simulink model "testemplanner_cs"  (R2020a)
settings: Solver=ode5  StartTime=0.0  StopTime=24  FixedStep=1/1000  RelTol=1e-3
PreLoadFcn:
  | mbxruntime.callbacks.PreLoadFcn(bdroot);
PostLoadFcn:
  | mbxruntime.callbacks.PostLoadFcn(bdroot);
InitFcn:
  | mbxruntime.callbacks.InitFcn(bdroot);
StartFcn:
  | mbxruntime.callbacks.StartFcn(bdroot);
StopFcn:
  | mbxruntime.callbacks.StopFcn(bdroot);
model workspace (MAT data in the model file):
  mbox_table : object (value not decoded)
  model_closed = 0
  sim_status = 0
values from neighbouring files (symbols this model uses):
  c_factor = 43.75    [emplanner_init.m]
  cf = -175016    [emplanner_init.m]
  cr = -130634    [emplanner_init.m]
  global_path_x = [0.057304 1.05668625507 2.05480936558 3.05165624935 4.04722112279 5.04150235808 6.03449985569 7.02621407764 8.01664569183 9.00579544113 9.99366409523 10.9802524329 ... (3001 elements, 3001x1)]    [global_path.mat]
  global_path_y = [8.29 8.29 8.29 8.29 8.29 8.29 8.29 8.29 8.29 8.29 8.29 8.29 ... (3001 elements, 3001x1)]    [global_path.mat]
  KD_PID_distance = 0.0    (= 0)    [emplanner_init.m]
  KD_PID_speed = 0    [emplanner_init.m]
  KI_PID_distance = 0.0    (= 0)    [emplanner_init.m]
  KI_PID_speed = 0    [emplanner_init.m]
  KP_PID_distance = 0.5    [emplanner_init.m]
  KP_PID_speed = 1.8    [emplanner_init.m]
  la = 1.265    [emplanner_init.m]
  lb = 2.947-1.265    (= 1.682)    [emplanner_init.m]
  LQR_K1 = k(:,1)'    [emplanner_init.m]
  LQR_K2 = k(:,2)'    [emplanner_init.m]
  LQR_K3 = k(:,3)'    [emplanner_init.m]
  LQR_K4 = k(:,4)'    [emplanner_init.m]
  m = 2020    [emplanner_init.m]
  rack_displacement = [-39.14 , -37.2 , -35.29 , -33.43 , -31.6 , -29.81 , -28.06 , -26.34 , -24.66 ,      -23.01 , -21.38 , -19.79 , -18.23 , -16.69 , -15.18 , -13.7 , -12.23 , -10.8 , -9.38 , -7.98 ,     -6.61 , -5.25 , -3.91 , -2.59 , -1.29 , 0 , 1.27 , 2.54 , 3.78 , 5.02 , 6.24 , 7.46 , 8.66 ,      9.86 , 11.05 , 12.24 , 13.41 , 14.59 , 15.76 , 16.92 , 18.09 , 19.25 , 20.42 , 21.59 , 22.76 ,      23.93 , 25.11 , 26 ...(+26 chars)    [emplanner_init.m]
  right_wheel_ground = [-70 ,-67.2 , -64.4 , -61.6 , -58.8 , -56 , -53.2 , -50.4 , -47.6 , -44.8 , -42 ,      -39.2 , -36.4 , -33.6 , -30.8 , -28 , -25.2 , -22.4 , -19.6 , -16.8 , -14 , -11.2 , -8.4 , -5.6 ,      -2.8 , 0 , 2.8 , 5.6 , 8.4 , 11.2 , 14 , 16.8 , 19.6 , 22.4 , 25.2 , 28 , 30.8 , 33.6 , 36.4 ,      39.2 , 42 , 44.8 , 47.6 , 50.4 , 53.2 , 56 , 58.8 , 61.6 , 64.4 , 67.2 , 70 ]    [emplanner_init.m]
  vx_break_point = zeros(1,5000)    [emplanner_init.m]
undefined symbols (not defined in the file or in its folder): aubr, DiscIntNeverNeededParam, tablebr, vubr
libraries: PreScanSimulinkLibrary x9, Solver_SF x1, simulink_extras x1
(part 3 of 9)

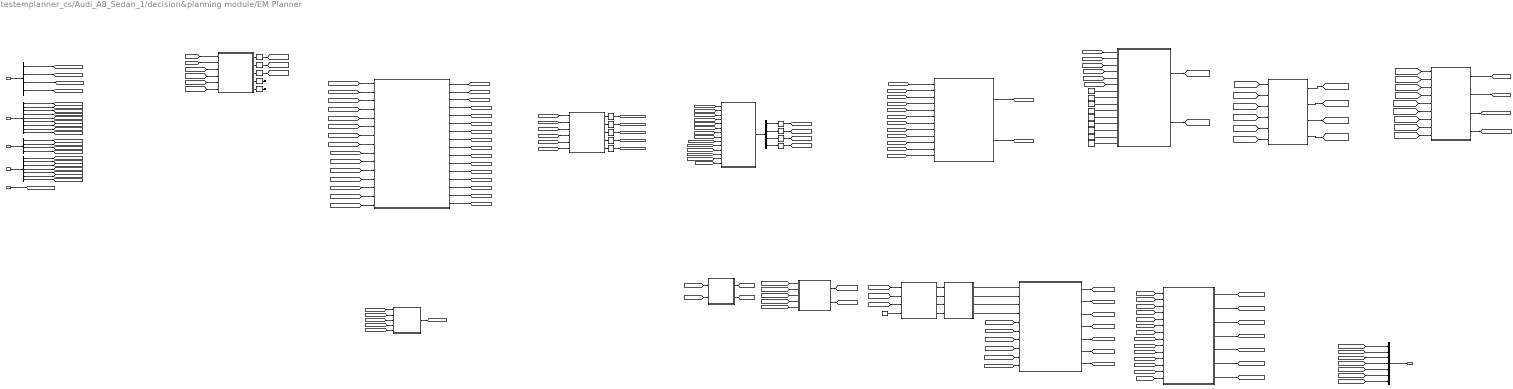
== system testemplanner_cs/Audi_A8_Sedan_1/decision&planning module/EM Planner ==
  note: 计算规划起点的投影点
  note: 模块输入整理，输入包括车辆当前位置、航向、速度、加速度信息。参考线信息，车辆在参考线上的投影点信息，感知获取的障碍物信息，当前的时间戳以及上一周期规划出的路径相关信息
  note: 找到规划路径起点，并通过拼接的方式进行平滑
  note: 计算index对应的s，并形成数组，方便进行查阅
  note: 进行动态规划所求路径的加密，以适应控制的需要
  note: 坐标变换，从Frenet坐标转换为直角坐标，进行控制
  note: 动态规划主函数
  note: 对障碍物进行筛选和投影
  note: 笛卡尔坐标转Frenet坐标
  note: 轨迹生成模块
  referenceline info : Inport
  location info : Inport  Port=2
  perception info : Inport  Port=3
  pre_planning info : Inport  Port=4
  current time : Inport  Port=5
  Bus Creator : BusCreator  Inputs=7
  Bus Selector : BusSelector  OutputSignals=referenceline_x,referenceline_y,path_heading,path_kappa
  Bus Selector1 : BusSelector  OutputSignals=host_x,host_y,host_heading_xy,host_vx,host_vy,host_yawrate,host_speed,host_ax,host_ay
  Bus Selector2 : BusSelector  OutputSignals=obs_x_set_gcs,obs_y_set_gcs,obs_velocity_set_gcs,obs_heading_set_gcs
  Bus Selector3 : BusSelector  OutputSignals=trajectory_x_gcs,trajectory_y_gcs,trajectory_heading_gcs,trajectory_kappa_gcs,trajectory_speed_gcs,trajectory_accel_gcs,trajectory_time_gcs
  Bus Selector5 : BusSelector  OutputSignals=s_set,l_set,dl_set,ddl_set
  Cartesian2Frenet1 : Subsystem
  Constant : Constant  Value=1e8
  Constant1 : Constant  Value=300
  Constant2 : Constant  Value=2000
  Constant3 : Constant  Value=10000
  Constant4 : Constant  Value=20
  Constant5 : Constant  Value=9
  Constant6 : Constant  Value=4
  Constant7 : Constant  Value=15
  Constant8 : Constant
  Constant9 : Constant  Value=8
  DP node generate1 : MATLAB Function  TreatAsAtomicUnit=on
  DP path1 : MATLAB Function  TreatAsAtomicUnit=on
  Frenet2Cart : MATLAB Function  TreatAsAtomicUnit=on
  Index to s : MATLAB Function  TreatAsAtomicUnit=on
  MATLAB Function1 : MATLAB Function  TreatAsAtomicUnit=on
  MATLAB Function5 : MATLAB Function  TreatAsAtomicUnit=on
  Selector{1..5,10..18} (14 alike) : Selector  InputPortWidth=128  IndexOptions=Index vector (dialog)  Indices=1  OutputSizes=1
  Terminator_5 : Terminator
  Terminator_6 : Terminator
  calc path length and map between point and s : MATLAB Function  TreatAsAtomicUnit=on
  calc plan start and stitch trajectory : MATLAB Function  TreatAsAtomicUnit=on
  calc speed planning start condition : MATLAB Function  TreatAsAtomicUnit=on
  increase st point count : MATLAB Function  TreatAsAtomicUnit=on
  obs1 : Subsystem
  path and speed merge : MATLAB Function  TreatAsAtomicUnit=on
  simple speed qp planning : MATLAB Function  TreatAsAtomicUnit=on
  stitch trajectory : MATLAB Function  TreatAsAtomicUnit=on
  EM Planner result : Outport
  wires:
  referenceline info/1 -> Bus Selector/1
  location info/1 -> Bus Selector1/1
  perception info/1 -> Bus Selector2/1
  pre_planning info/1 -> Bus Selector3/1
  current time/1 -> [current_time]
  Bus Selector3/1 -> [pre_trajectory_x_gcs]  "<trajectory_x_gcs>"
  Bus Selector3/2 -> [pre_trajectory_y_gcs]  "<trajectory_y_gcs>"
  Bus Selector3/3 -> [pre_trajectory_heading_gcs]  "<trajectory_heading_gcs>"
  Bus Selector3/4 -> [pre_trajectory_kappa_gcs]  "<trajectory_kappa_gcs>"
  Bus Selector3/5 -> [pre_trajectory_speed_gcs]  "<trajectory_speed_gcs>"
  Bus Selector3/6 -> [pre_trajectory_accel_gcs]  "<trajectory_accel_gcs>"
  Bus Selector3/7 -> [pre_trajectory_time]  "<trajectory_time_gcs>"
  Bus Selector2/1 -> [obs_x_set_gcs]  "<obs_x_set_gcs>"
  Bus Selector2/2 -> [obs_y_set_gcs]  "<obs_y_set_gcs>"
  Bus Selector2/3 -> [obs_velocity_set_gcs]  "<obs_velocity_set_gcs>"
  Bus Selector2/4 -> [obs_heading_set_gcs]  "<obs_heading_set_gcs>"
  Bus Selector1/1 -> [host_x]  "<host_x>"
  Bus Selector1/2 -> [host_y]  "<host_y>"
  Bus Selector1/3 -> [host_heading_xy]  "<host_heading_xy>"
  Bus Selector1/4 -> [host_vx_vcs]  "<host_vx>"
  Bus Selector1/5 -> [host_vy_vcs]  "<host_vy>"
  Bus Selector1/6 -> [host_yawrate]  "<host_yawrate>"
  Bus Selector1/7 -> [host_speed]  "<host_speed>"
  Bus Selector1/8 -> [host_ax_vcs]  "<host_ax>"
  Bus Selector1/9 -> [host_ay_vcs]  "<host_ay>"
  Bus Selector/1 -> [referenceline_x]  "<referenceline_x>"
  Bus Selector/2 -> [referenceline_y]  "<referenceline_y>"
  Bus Selector/3 -> [referenceline_heading]  "<path_heading>"
  Bus Selector/4 -> [referenceline_kappa]  "<path_kappa>"
  [referenceline_x] -> Index to s/1(path_x)
  [referenceline_y] -> Index to s/2(path_y)
  [origin_x] -> Index to s/3(origin_point_x)
  [origin_y] -> Index to s/4(origin_point_y)
  [origin_match_point_index] -> Index to s/5(origin_match_point_index)
  Index to s/1(index2s) -> [index2s]
  MATLAB Function1/5(proj_kappa_set) -> Selector5/1
  MATLAB Function1/3(proj_y_set) -> Selector3/1
  MATLAB Function1/1(match_point_index_set) -> Selector1/1
  MATLAB Function1/4(proj_heading_set) -> Selector4/1
  MATLAB Function1/2(proj_x_set) -> Selector2/1
  [plan_start_x_gcs] -> MATLAB Function1/1(x_set)
  [plan_start_y_gcs] -> MATLAB Function1/2(y_set)
  [referenceline_x] -> MATLAB Function1/3(frenet_path_x)
  [referenceline_y] -> MATLAB Function1/4(frenet_path_y)
  [referenceline_heading] -> MATLAB Function1/5(frenet_path_heading)
  [referenceline_kappa] -> MATLAB Function1/6(frenet_path_kappa)
  Selector1/1 -> [plan_start_match_point_index]
  Selector2/1 -> [plan_start_proj_x]
  Selector3/1 -> [plan_start_proj_y]
  Selector4/1 -> [plan_start_proj_heading]
  Selector5/1 -> [plan_start_proj_kappa]
  [static_obs_s_set] -> DP path1/1(obs_s_set)
  [static_obs_l_set] -> DP path1/2(obs_l_set)
  [plan_start_s] -> DP path1/3(plan_start_s)
  [plan_start_l] -> DP path1/4(plan_start_l)
  [plan_start_dl] -> DP path1/5(plan_start_dl)
  [plan_start_ddl] -> DP path1/6(plan_start_ddl)
  Constant/1 -> DP path1/7(w_collision_cost)
  Constant1/1 -> DP path1/8(w_smooth_dl_cost)
  Constant2/1 -> DP path1/9(w_smooth_ddl_cost)
  Constant3/1 -> DP path1/10(w_smooth_dddl_cost)
  Constant4/1 -> DP path1/11(w_ref_cost)
  Constant5/1 -> DP path1/12(row)
  Constant6/1 -> DP path1/13(col)
  Constant7/1 -> DP path1/14(sample_s)
  Constant8/1 -> DP path1/15(sample_l)
  path and speed merge/7(trajectory_time) -> [trajectory_time]
  path and speed merge/1(trajectory_x) -> [trajectory_x]
  [trajectory_speed] -> stitch trajectory/5(trajectory_speed)
  path and speed merge/4(trajectory_kappa) -> [trajectory_kappa]
  [plan_start_vy_gcs] -> calc speed planning start condition/2(plan_start_vy)
  [stitch_time] -> stitch trajectory/14(stitch_time)
  calc path length and map between point and s/2(path_s) -> [path_s]
  [plan_start_heading_gcs] -> calc speed planning start condition/5(plan_start_heading)
  simple speed qp planning/2(s_dot_init) -> increase st point count/2(s_dot_init)
  Bus Creator/1 -> EM Planner result/1
  simple speed qp planning/1(s_init) -> increase st point count/1(s_init)
  [trajectory_x_final] -> Bus Creator/1  "trajectory_x_gcs"
  stitch trajectory/4(trajectory_kappa_final) -> [trajectory_kappa_final]
  [plan_start_ax_gcs] -> calc speed planning start condition/3(plan_start_ax)
  calc speed planning start condition/1(plan_start_s_dot) -> [plan_start_s_dot]
  [plan_start_ay_gcs] -> calc speed planning start condition/4(plan_start_ay)
  [stitch_speed_gcs] -> stitch trajectory/12(stitch_speed)
  [trajectory_time_final] -> Bus Creator/7  "trajectory_time_gcs"
  Constant9/1 -> simple speed qp planning/4(recommend_T)
  [stitch_x_gcs] -> stitch trajectory/8(stitch_x)
  stitch trajectory/1(trajectory_x_final) -> [trajectory_x_final]
  [trajectory_accel_final] -> Bus Creator/6  "trajectory_accel_gcs"
  [stitch_heading_gcs] -> stitch trajectory/10(stitch_heading)
  [trajectory_speed_final] -> Bus Creator/5  "trajectory_speed_gcs"
  [stitch_y_gcs] -> stitch trajectory/9(stitch_y)
  stitch trajectory/6(trajectory_accel_final) -> [trajectory_accel_final]
  [plan_start_s_dot2] -> simple speed qp planning/2(plan_start_s_dot2)
  increase st point count/3(s_dot2) -> path and speed merge/3(s_dot2)
  [plan_start_vx_gcs] -> calc speed planning start condition/1(plan_start_vx)
  [trajectory_heading_final] -> Bus Creator/3  "trajectory_heading_gcs"
  [trajectory_accel] -> stitch trajectory/6(trajectory_accel)
  [trajectory_kappa] -> stitch trajectory/4(trajectory_kappa)
  stitch trajectory/7(trajectory_time_final) -> [trajectory_time_final]
  [trajectory_x_init] -> path and speed merge/7(trajectory_x_init)
  stitch trajectory/2(trajectory_y_final) -> [trajectory_y_final]
  increase st point count/2(s_dot) -> path and speed merge/2(s_dot)
  stitch trajectory/3(trajectory_heading_final) -> [trajectory_heading_final]
  [trajectory_kappa_final] -> Bus Creator/4  "trajectory_kappa_gcs"
  [plan_start_s_dot] -> simple speed qp planning/1(plan_start_s_dot)
  path and speed merge/3(trajectory_heading) -> [trajectory_heading]
  simple speed qp planning/3(s_dot2_init) -> increase st point count/3(s_dot2_init)
  stitch trajectory/5(trajectory_speed_final) -> [trajectory_speed_final]
  [trajectory_y_final] -> Bus Creator/2  "trajectory_y_gcs"
  [trajectory_y] -> stitch trajectory/2(trajectory_y)
  calc path length and map between point and s/1(path_s_end) -> [path_s_end]
  calc speed planning start condition/2(plan_start_s_dot2) -> [plan_start_s_dot2]
  [trajectory_kappa_init] -> path and speed merge/10(trajectory_kappa_init)
  [stitch_accel_gcs] -> stitch trajectory/13(stitch_accel)
  increase st point count/1(s) -> path and speed merge/1(s)
  [trajectory_x] -> stitch trajectory/1(trajectory_x)
  [trajectory_y_init] -> calc path length and map between point and s/2(trajectory_y)
  [path_s_end] -> simple speed qp planning/3(s_end)
  path and speed merge/6(trajectory_accel) -> [trajectory_accel]
  [stitch_kappa_gcs] -> stitch trajectory/11(stitch_kappa)
  increase st point count/4(relative_time) -> path and speed merge/4(relative_time)
  [path_s] -> path and speed merge/6(path_s)
  path and speed merge/2(trajectory_y) -> [trajectory_y]
  [trajectory_heading_init] -> path and speed merge/9(trajectory_heading_init)
  [plan_start_time] -> path and speed merge/5(current_time)
  path and speed merge/5(trajectory_speed) -> [trajectory_speed]
  simple speed qp planning/4(relative_time_init) -> increase st point count/4(relative_time_init)
  [trajectory_y_init] -> path and speed merge/8(trajectory_y_init)
  [trajectory_time] -> stitch trajectory/7(trajectory_time)
  [trajectory_heading] -> stitch trajectory/3(trajectory_heading)
  [trajectory_x_init] -> calc path length and map between point and s/1(trajectory_x)
  DP path1/1(dp_path_s) -> [dp_path_s_init]
  DP path1/2(dp_path_l) -> [dp_path_l_init]
  [dp_path_s_final] -> Frenet2Cart/1(s_set)
  [dp_path_l_final] -> Frenet2Cart/2(l_set)
  [dp_path_dl_final] -> Frenet2Cart/3(dl_set)
  [dp_path_ddl_final] -> Frenet2Cart/4(ddl_set)
  [index2s] -> Frenet2Cart/9(index2s)
  [referenceline_x] -> Frenet2Cart/5(frenet_s)
  [referenceline_y] -> Frenet2Cart/6(frenet_l)
  [referenceline_heading] -> Frenet2Cart/7(frenet_heading)
  [referenceline_kappa] -> Frenet2Cart/8(frenet_kappa)
  Frenet2Cart/1(x_set) -> [trajectory_x_init]
  Frenet2Cart/2(y_set) -> [trajectory_y_init]
  Frenet2Cart/3(heading_set) -> [trajectory_heading_init]
  Frenet2Cart/4(kappa_set) -> [trajectory_kappa_init]
  MATLAB Function5/5(proj_kappa_set) -> Selector14/1
  [host_y] -> MATLAB Function5/2(y_set)
  MATLAB Function5/1(match_point_index_set) -> Selector10/1
  Selector13/1 -> Terminator_5/1
  Selector14/1 -> Terminator_6/1
  Selector11/1 -> [origin_x]
  MATLAB Function5/2(proj_x_set) -> Selector11/1
  Selector10/1 -> [origin_match_point_index]
  MATLAB Function5/3(proj_y_set) -> Selector12/1
  [referenceline_y] -> MATLAB Function5/4(frenet_path_y)
  [referenceline_x] -> MATLAB Function5/3(frenet_path_x)
  [referenceline_heading] -> MATLAB Function5/5(frenet_path_heading)
  MATLAB Function5/4(proj_heading_set) -> Selector13/1
  [referenceline_kappa] -> MATLAB Function5/6(frenet_path_kappa)
  Selector12/1 -> [origin_y]
  [host_x] -> MATLAB Function5/1(x_set)
  [index2s] -> Cartesian2Frenet1/14(index2s)
  Selector18/1 -> [plan_start_ddl]
  Selector17/1 -> [plan_start_dl]
  Selector16/1 -> [plan_start_l]
  Selector15/1 -> [plan_start_s]
  Bus Selector5/1 -> Selector15/1  "<s_set>"
  Bus Selector5/2 -> Selector16/1  "<l_set>"
  Bus Selector5/3 -> Selector17/1  "<dl_set>"
  Bus Selector5/4 -> Selector18/1  "<ddl_set>"
  Cartesian2Frenet1/1(Cartesian2FrenetOut) -> Bus Selector5/1
  [plan_start_proj_kappa] -> Cartesian2Frenet1/13(proj_kappa_set)
  [plan_start_proj_heading] -> Cartesian2Frenet1/12(proj_heading_set)
  [plan_start_proj_y] -> Cartesian2Frenet1/11(proj_y_set)
  [plan_start_proj_x] -> Cartesian2Frenet1/10(proj_x_set)
  [plan_start_match_point_index] -> Cartesian2Frenet1/9(proj_match_point_index_set)
  [referenceline_y] -> Cartesian2Frenet1/8(frenet_path_y)
  [referenceline_x] -> Cartesian2Frenet1/7(frenet_path_x)
  [plan_start_ay_gcs] -> Cartesian2Frenet1/6(ay_set)
  [plan_start_ax_gcs] -> Cartesian2Frenet1/5(ax_set)
  [plan_start_vy_gcs] -> Cartesian2Frenet1/4(vy_set)
  [plan_start_vx_gcs] -> Cartesian2Frenet1/3(vx_set)
  [plan_start_x_gcs] -> Cartesian2Frenet1/1(x_set)
  [plan_start_y_gcs] -> Cartesian2Frenet1/2(y_set)
  DP node generate1/4(dp_path_ddl_final) -> [dp_path_ddl_final]
  DP node generate1/3(dp_path_dl_final) -> [dp_path_dl_final]
  DP node generate1/2(dp_path_l_final) -> [dp_path_l_final]
  DP node generate1/1(dp_path_s_final) -> [dp_path_s_final]
  [plan_start_dl] -> DP node generate1/5(plan_start_dl)
  [plan_start_ddl] -> DP node generate1/6(plan_start_ddl)
  [plan_start_l] -> DP node generate1/4(plan_start_l)
  [plan_start_s] -> DP node generate1/3(plan_start_s)
  [dp_path_l_init] -> DP node generate1/2(dp_path_l_init)
  [dp_path_s_init] -> DP node generate1/1(dp_path_s_init)
  [pre_trajectory_x_gcs] -> calc plan start and stitch trajectory/8(pre_trajectory_x)
  [pre_trajectory_y_gcs] -> calc plan start and stitch trajectory/9(pre_trajectory_y)
  [host_heading_xy] -> calc plan start and stitch trajectory/3(host_heading_xy)
  [host_y] -> calc plan start and stitch trajectory/2(host_y)
  [pre_trajectory_heading_gcs] -> calc plan start and stitch trajectory/10(pre_trajectory_heading)
  [host_vx_vcs] -> calc plan start and stitch trajectory/4(host_vx)
  [host_x] -> calc plan start and stitch trajectory/1(host_x)
  [pre_trajectory_kappa_gcs] -> calc plan start and stitch trajectory/11(pre_trajectory_kappa)
  [host_vy_vcs] -> calc plan start and stitch trajectory/5(host_vy)
  [pre_trajectory_speed_gcs] -> calc plan start and stitch trajectory/12(pre_trajectory_velocity)
  [host_ax_vcs] -> calc plan start and stitch trajectory/6(host_ax)
  [pre_trajectory_accel_gcs] -> calc plan start and stitch trajectory/13(pre_trajectory_accelerate)
  [host_ay_vcs] -> calc plan start and stitch trajectory/7(host_ay)
  [pre_trajectory_time] -> calc plan start and stitch trajectory/14(pre_trajectory_time)
  [current_time] -> calc plan start and stitch trajectory/15(current_time)
  calc plan start and stitch trajectory/5(plan_start_vx) -> [plan_start_vx_gcs]
  calc plan start and stitch trajectory/6(plan_start_vy) -> [plan_start_vy_gcs]
  calc plan start and stitch trajectory/4(plan_start_kappa) -> [plan_start_kappa_gcs]
  calc plan start and stitch trajectory/7(plan_start_ax) -> [plan_start_ax_gcs]
  calc plan start and stitch trajectory/3(plan_start_heading) -> [plan_start_heading_gcs]
  calc plan start and stitch trajectory/8(plan_start_ay) -> [plan_start_ay_gcs]
  calc plan start and stitch trajectory/2(plan_start_y) -> [plan_start_y_gcs]
  calc plan start and stitch trajectory/9(plan_start_time) -> [plan_start_time]
  calc plan start and stitch trajectory/1(plan_start_x) -> [plan_start_x_gcs]
  calc plan start and stitch trajectory/10(stitch_x) -> [stitch_x_gcs]
  calc plan start and stitch trajectory/11(stitch_y) -> [stitch_y_gcs]
  calc plan start and stitch trajectory/12(stitch_heading) -> [stitch_heading_gcs]
  calc plan start and stitch trajectory/13(stitch_kappa) -> [stitch_kappa_gcs]
  calc plan start and stitch trajectory/14(stitch_velocity) -> [stitch_speed_gcs]
  calc plan start and stitch trajectory/15(stitch_accelerate) -> [stitch_accel_gcs]
  calc plan start and stitch trajectory/16(stitch_time) -> [stitch_time]
  [obs_y_set_gcs] -> obs1/5(obs_y_set_gcs)
  [obs_x_set_gcs] -> obs1/4(obs_x_set_gcs)
  [obs_velocity_set_gcs] -> obs1/6(obs_velocity_set_gcs)
  [host_heading_xy] -> obs1/3(host_heading_xy)
  [obs_heading_set_gcs] -> obs1/7(obs_heading_set_gcs)
  [host_y] -> obs1/2(host_y)
  [referenceline_x] -> obs1/8(referenceline_x)
  [host_x] -> obs1/1(host_x)
  [referenceline_y] -> obs1/9(referenceline_y)
  [referenceline_heading] -> obs1/10(referenceline_heading)
  [referenceline_kappa] -> obs1/11(referenceline_kappa)
  [index2s] -> obs1/12(index2s)
  obs1/1(static_obs_s_set) -> [static_obs_s_set]
  obs1/2(static_obs_l_set) -> [static_obs_l_set]

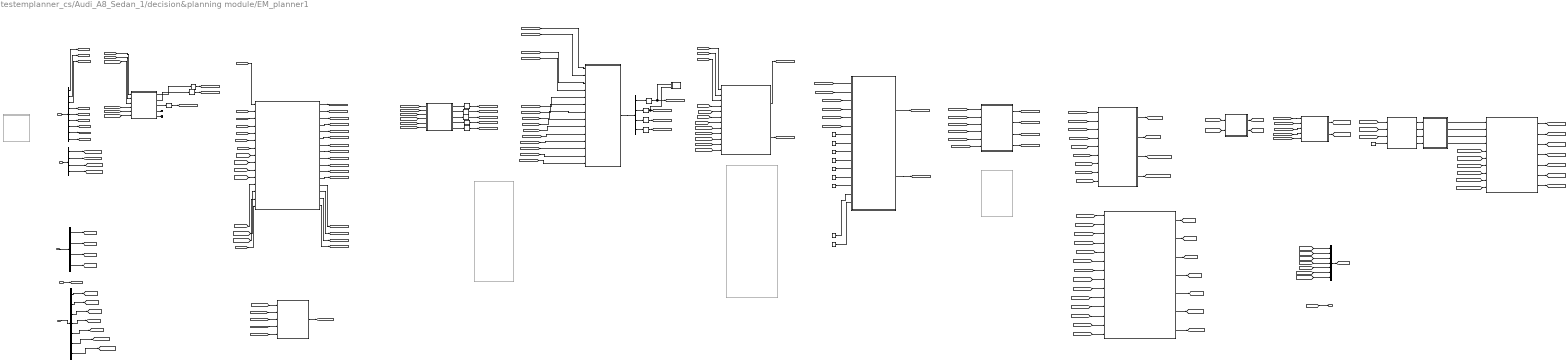
== system testemplanner_cs/Audi_A8_Sedan_1/decision&planning module/EM_planner1 ==
  note: 轨迹生成模块
  note: 坐标变换，从Frenet坐标转换为直角坐标，进行控制
  note: 进行动态规划所求路径的加密，以适应控制的需要
  note: 动态规划主函数
  note: 对障碍物进行筛选和投影
  note: 规划起点进行投影
  note: 计算规划起点的投影点
  note: 计算index对应的s，并形成数组，方便进行查阅
  note: 找到规划路径起点，并通过拼接的方式进行平滑
  note: 模块输入整理，输入包括车辆当前位置、航向、速度、加速度信息。参考线信息，车辆在参考线上的投影点信息，感知获取的障碍物信息，当前的时间戳以及上一周期规划出的路径相关信息
  Location_info : Inport
  referenceline_info : Inport  Port=2
  perceptiong_result : Inport  Port=3
  current_time : Inport  Port=4
  pre_planning_result : Inport  Port=5
  Bus Creator1 : BusCreator  Inputs=7
  Bus Selector : BusSelector  OutputSignals=host_x,host_y,host_heading_xy,host_vx,host_vy,host_yawrate,host_speed,host_ax,host_ay
  Bus Selector1 : BusSelector  OutputSignals=referenceline_x,referenceline_y,path_heading,path_kappa
  Bus Selector2 : BusSelector  OutputSignals=obs_x_set_gcs,obs_y_set_gcs,obs_velocity_set_gcs,obs_heading_set_gcs
  Bus Selector3 : BusSelector  OutputSignals=trajectory_x_final[m],trajectory_y_final[m],trajectory_heading_final[rad],trajectory_kappa_final[1/m],trajectory_velocity_final[m/s],trajectory_accelerate_final[m/s^2],trajectory_time_final[m/s^2]
  Bus Selector4 : BusSelector  OutputSignals=s_set,l_set,dl_set,ddl_set
  Cart2Frenet1 : Subsystem  Commented=on
  Cartesian2Frenet : Subsystem
  Constant9 : Constant  Value=8
  DP node generate : MATLAB Function  TreatAsAtomicUnit=on
  DP node generate1 : MATLAB Function  Commented=on  TreatAsAtomicUnit=on
  DP path1 : MATLAB Function  Commented=on  TreatAsAtomicUnit=on
  Frenet2Cart : MATLAB Function  TreatAsAtomicUnit=on
  Index to s : MATLAB Function  TreatAsAtomicUnit=on
  MATLAB Function : MATLAB Function  TreatAsAtomicUnit=on
  MATLAB Function1 : MATLAB Function  TreatAsAtomicUnit=on
  MATLAB Function2 : MATLAB Function  TreatAsAtomicUnit=on
  Selector{,1..11} (12 alike) : Selector  InputPortWidth=128  IndexOptions=Index vector (dialog)  Indices=[1]  OutputSizes=1
  Terminator_1 : Terminator
  Terminator_2 : Terminator
  calc path length and map between point and s : MATLAB Function  TreatAsAtomicUnit=on
  calc plan start and stitch trajectory : MATLAB Function  TreatAsAtomicUnit=on
  calc speed planning start condition : MATLAB Function  TreatAsAtomicUnit=on
  col : Constant  Value=4
  general fast algorithm to find projection point info3 : MATLAB Function  Commented=on  TreatAsAtomicUnit=on
  increase st point count : MATLAB Function  TreatAsAtomicUnit=on
  obs : Subsystem
  path and speed merge : MATLAB Function  TreatAsAtomicUnit=on
  path decision with dynamic planning(dp) : MATLAB Function  TreatAsAtomicUnit=on
  row : Constant  Value=9
  sample_l : Constant
  sample_s : Constant  Value=15
  simple speed qp planning : MATLAB Function  TreatAsAtomicUnit=on
  stitch trajectory : MATLAB Function  TreatAsAtomicUnit=on
  w_collision : Constant  Value=10000
  w_ref : Constant  Value=2000
  w_smooth_dddl : Constant  Value=20
  w_smooth_ddl : Constant  Value=1e8
  w_smooth_dl : Constant  Value=300
  EMplanner_result : Outport
  wires:
  [ddl_set] -> path decision with dynamic planning(dp)/6(plan_start_dll)
  [dl_set] -> path decision with dynamic planning(dp)/5(plan_start_dl)
  w_ref/1 -> path decision with dynamic planning(dp)/11(w_cost_ref)
  w_smooth_dddl/1 -> path decision with dynamic planning(dp)/10(w_cost_smooth_dddl)
  w_smooth_ddl/1 -> path decision with dynamic planning(dp)/9(w_cost_smooth_ddl)
  w_smooth_dl/1 -> path decision with dynamic planning(dp)/8(w_cost_smooth_dl)
  w_collision/1 -> path decision with dynamic planning(dp)/7(w_cost_collision)
  calc path length and map between point and s/1(path_s_end) -> [path_s_end]
  [trajectory_kappa_init] -> path and speed merge/10(trajectory_kappa_init)
  [trajectory_x_init] -> calc path length and map between point and s/1(trajectory_x)
  calc path length and map between point and s/2(path_s) -> [path_s]
  path and speed merge/5(trajectory_speed) -> [trajectory_speed]
  [plan_start_s_dot] -> simple speed qp planning/1(plan_start_s_dot)
  [path_s_end] -> simple speed qp planning/3(s_end)
  simple speed qp planning/1(s_init) -> increase st point count/1(s_init)
  [trajectory_y_init] -> calc path length and map between point and s/2(trajectory_y)
  increase st point count/3(s_dot2) -> path and speed merge/3(s_dot2)
  [plan_start_vy] -> calc speed planning start condition/2(plan_start_vy)
  path and speed merge/3(trajectory_heading) -> [trajectory_heading]
  path and speed merge/4(trajectory_kappa) -> [trajectory_kappa]
  Constant9/1 -> simple speed qp planning/4(recommend_T)
  [trajectory_heading_init] -> path and speed merge/9(trajectory_heading_init)
  simple speed qp planning/2(s_dot_init) -> increase st point count/2(s_dot_init)
  path and speed merge/2(trajectory_y) -> [trajectory_y]
  calc speed planning start condition/2(plan_start_s_dot2) -> [plan_start_s_dot2]
  [plan_start_time] -> path and speed merge/5(current_time)
  calc speed planning start condition/1(plan_start_s_dot) -> [plan_start_s_dot]
  [plan_start_ax] -> calc speed planning start condition/3(plan_start_ax)
  path and speed merge/1(trajectory_x) -> [trajectory_x]
  increase st point count/1(s) -> path and speed merge/1(s)
  increase st point count/4(relative_time) -> path and speed merge/4(relative_time)
  [plan_start_ay] -> calc speed planning start condition/4(plan_start_ay)
  [trajectory_y_init] -> path and speed merge/8(trajectory_y_init)
  path and speed merge/6(trajectory_accel) -> [trajectory_accel]
  [path_s] -> path and speed merge/6(path_s)
  path and speed merge/7(trajectory_time) -> [trajectory_time]
  simple speed qp planning/4(relative_time_init) -> increase st point count/4(relative_time_init)
  [plan_start_s_dot2] -> simple speed qp planning/2(plan_start_s_dot2)
  increase st point count/2(s_dot) -> path and speed merge/2(s_dot)
  [trajectory_x_init] -> path and speed merge/7(trajectory_x_init)
  simple speed qp planning/3(s_dot2_init) -> increase st point count/3(s_dot2_init)
  [plan_start_vx] -> calc speed planning start condition/1(plan_start_vx)
  [plan_start_heading] -> calc speed planning start condition/5(plan_start_heading)
  stitch trajectory/6(trajectory_accel_final) -> [trajectory_accelerate_final]
  stitch trajectory/5(trajectory_speed_final) -> [trajectory_velocity_final]
  stitch trajectory/4(trajectory_kappa_final) -> [trajectory_kappa_final]
  stitch trajectory/7(trajectory_time_final) -> [trajectory_time_final]
  stitch trajectory/3(trajectory_heading_final) -> [trajectory_heading_final]
  stitch trajectory/2(trajectory_y_final) -> [trajectory_y_final]
  stitch trajectory/1(trajectory_x_final) -> [trajectory_x_final]
  [stitch_time] -> stitch trajectory/14(stitch_time)
  [stitch_accelerate] -> stitch trajectory/13(stitch_accel)
  [stitch_kappa] -> stitch trajectory/11(stitch_kappa)
  [stitch_heading] -> stitch trajectory/10(stitch_heading)
  [stitch_velocity] -> stitch trajectory/12(stitch_speed)
  [stitch_y] -> stitch trajectory/9(stitch_y)
  [stitch_x] -> stitch trajectory/8(stitch_x)
  [trajectory_time] -> stitch trajectory/7(trajectory_time)
  [trajectory_accel] -> stitch trajectory/6(trajectory_accel)
  [trajectory_speed] -> stitch trajectory/5(trajectory_speed)
  [trajectory_kappa] -> stitch trajectory/4(trajectory_kappa)
  [trajectory_heading] -> stitch trajectory/3(trajectory_heading)
  [trajectory_y] -> stitch trajectory/2(trajectory_y)
  [trajectory_x] -> stitch trajectory/1(trajectory_x)
  Frenet2Cart/4(kappa_set) -> [trajectory_kappa_init]
  Frenet2Cart/3(heading_set) -> [trajectory_heading_init]
  Frenet2Cart/2(y_set) -> [trajectory_y_init]
  Frenet2Cart/1(x_set) -> [trajectory_x_init]
  [dp_path_s_final] -> Frenet2Cart/1(s_set)
  [dp_path_l_final] -> Frenet2Cart/2(l_set)
  [dp_path_dl_final] -> Frenet2Cart/3(dl_set)
  [dp_path_ddl_final] -> Frenet2Cart/4(ddl_set)
  [referenceline_x] -> Frenet2Cart/5(frenet_s)
  [referenceline_y] -> Frenet2Cart/6(frenet_l)
  [referenceline_heading] -> Frenet2Cart/7(frenet_heading)
  [referenceline_kappa] -> Frenet2Cart/8(frenet_kappa)
  [index2s] -> Frenet2Cart/9(index2s)
  DP node generate/2(dp_path_l_final) -> [dp_path_l_final]
  DP node generate/3(dp_path_dl_final) -> [dp_path_dl_final]
  DP node generate/4(dp_path_ddl_final) -> [dp_path_ddl_final]
  DP node generate/1(dp_path_s_final) -> [dp_path_s_final]
  [ddl_set] -> DP node generate/6(plan_start_ddl)
  [dl_set] -> DP node generate/5(plan_start_dl)
  [l_set] -> DP node generate/4(plan_start_l)
  [s_set] -> DP node generate/3(plan_start_s)
  [dp_path_l_init_set] -> DP node generate/2(dp_path_l_init)
  [dp_path_s_init_set] -> DP node generate/1(dp_path_s_init)
  path decision with dynamic planning(dp)/2(dp_path_l) -> [dp_path_l_init_set]
  path decision with dynamic planning(dp)/1(dp_path_s) -> [dp_path_s_init_set]
  sample_l/1 -> path decision with dynamic planning(dp)/15(sample_l)
  sample_s/1 -> path decision with dynamic planning(dp)/14(sample_s)
  row/1 -> path decision with dynamic planning(dp)/13(col)
  col/1 -> path decision with dynamic planning(dp)/12(row)
  [l_set] -> path decision with dynamic planning(dp)/4(plan_start_l)
  [s_set] -> path decision with dynamic planning(dp)/3(plan_start_s)
  [static_obs_l_set] -> path decision with dynamic planning(dp)/2(obs_l_set)
  [static_obs_s_set] -> path decision with dynamic planning(dp)/1(obs_s_set)
  obs/2(static_obs_l_set) -> [static_obs_l_set]
  obs/1(static_obs_s_set) -> [static_obs_s_set]
  Selector11/1 -> [ddl_set]
  Selector10/1 -> [dl_set]
  Selector9/1 -> [l_set], MATLAB Function/2(l)
  Selector8/1 -> [s_set], MATLAB Function/1(s)
  Bus Selector4/4 -> Selector11/1  "<ddl_set>"
  Bus Selector4/3 -> Selector10/1  "<dl_set>"
  Bus Selector4/2 -> Selector9/1  "<l_set>"
  Bus Selector4/1 -> Selector8/1  "<s_set>"
  Cartesian2Frenet/1(Cartesian2FrenetOut) -> Bus Selector4/1
  [index2s] -> obs/12(index2s)
  [referenceline_kappa] -> obs/11(referenceline_kappa)
  [referenceline_heading] -> obs/10(referenceline_heading)
  [referenceline_y] -> obs/9(referenceline_y)
  [referenceline_x] -> obs/8(referenceline_x)
  [obs_heading_set_gcs] -> obs/7(obs_heading_set_gcs)
  [obs_velocity_set_gcs] -> obs/6(obs_velocity_set_gcs)
  [obs_y_set_gcs] -> obs/5(obs_y_set_gcs)
  [obs_x_set_gcs] -> obs/4(obs_x_set_gcs)
  [host_y] -> obs/2(host_y)
  [host_heading_xy] -> obs/3(host_heading_xy)
  [host_x] -> obs/1(host_x)
  [plan_start_proj_kappa] -> Cartesian2Frenet/14(index2s)
  [plan_start_proj_heading] -> Cartesian2Frenet/13(proj_kappa_set)
  [plan_start_proj_y] -> Cartesian2Frenet/12(proj_heading_set)
  [plan_start_proj_x] -> Cartesian2Frenet/11(proj_y_set)
  [plan_start_match_point_index] -> Cartesian2Frenet/10(proj_x_set)
  [index2s] -> Cartesian2Frenet/9(proj_match_point_index_set)
  [referenceline_y] -> Cartesian2Frenet/8(frenet_path_y)
  [referenceline_x] -> Cartesian2Frenet/7(frenet_path_x)
  [plan_start_ay] -> Cartesian2Frenet/6(ay_set)
  [plan_start_ax] -> Cartesian2Frenet/5(ax_set)
  [plan_start_vy] -> Cartesian2Frenet/4(vy_set)
  [plan_start_vx] -> Cartesian2Frenet/3(vx_set)
  [plan_start_y] -> Cartesian2Frenet/2(y_set)
  [plan_start_x] -> Cartesian2Frenet/1(x_set)
  Selector7/1 -> [plan_start_proj_kappa]
  Selector6/1 -> [plan_start_proj_heading]
  MATLAB Function2/4(proj_heading_set) -> Selector6/1
  [referenceline_kappa] -> MATLAB Function2/6(frenet_path_kappa)
  MATLAB Function2/2(proj_x_set) -> Selector4/1
  [plan_start_x] -> MATLAB Function2/1(x_set)
  MATLAB Function2/1(match_point_index_set) -> Selector3/1
  [plan_start_y] -> MATLAB Function2/2(y_set)
  [referenceline_x] -> MATLAB Function2/3(frenet_path_x)
  MATLAB Function2/5(proj_kappa_set) -> Selector7/1
  [referenceline_heading] -> MATLAB Function2/5(frenet_path_heading)
  [referenceline_y] -> MATLAB Function2/4(frenet_path_y)
  MATLAB Function2/3(proj_y_set) -> Selector5/1
  Selector3/1 -> [plan_start_match_point_index]
  Selector4/1 -> [plan_start_proj_x]
  Selector5/1 -> [plan_start_proj_y]
  Index to s/1(index2s) -> [index2s]
  [origin_x] -> Index to s/3(origin_point_x)
  [origin_y] -> Index to s/4(origin_point_y)
  [origin_match_point_index] -> Index to s/5(origin_match_point_index)
  [referenceline_y] -> Index to s/2(path_y)
  [referenceline_x] -> Index to s/1(path_x)
  calc plan start and stitch trajectory/16(stitch_time) -> [stitch_time]
  calc plan start and stitch trajectory/15(stitch_accelerate) -> [stitch_accelerate]
  calc plan start and stitch trajectory/14(stitch_velocity) -> [stitch_velocity]
  calc plan start and stitch trajectory/13(stitch_kappa) -> [stitch_kappa]
  calc plan start and stitch trajectory/12(stitch_heading) -> [stitch_heading]
  calc plan start and stitch trajectory/11(stitch_y) -> [stitch_y]
  calc plan start and stitch trajectory/10(stitch_x) -> [stitch_x]
  calc plan start and stitch trajectory/9(plan_start_time) -> [plan_start_time]
  calc plan start and stitch trajectory/8(plan_start_ay) -> [plan_start_ay]
  calc plan start and stitch trajectory/7(plan_start_ax) -> [plan_start_ax]
  calc plan start and stitch trajectory/6(plan_start_vy) -> [plan_start_vy]
  calc plan start and stitch trajectory/5(plan_start_vx) -> [plan_start_vx]
  calc plan start and stitch trajectory/4(plan_start_kappa) -> [plan_start_kappa]
  calc plan start and stitch trajectory/3(plan_start_heading) -> [plan_start_heading]
  calc plan start and stitch trajectory/2(plan_start_y) -> [plan_start_y]
  calc plan start and stitch trajectory/1(plan_start_x) -> [plan_start_x]
  [current_time] -> calc plan start and stitch trajectory/15(current_time)
  [pre_trajectory_y] -> calc plan start and stitch trajectory/9(pre_trajectory_y)
  [pre_trajectory_time] -> calc plan start and stitch trajectory/14(pre_trajectory_time)
  [pre_trajectory_accelerate] -> calc plan start and stitch trajectory/13(pre_trajectory_accelerate)
  [pre_trajectory_velocity] -> calc plan start and stitch trajectory/12(pre_trajectory_velocity)
  [pre_trajectory_kappa] -> calc plan start and stitch trajectory/11(pre_trajectory_kappa)
  [pre_trajectory_heading] -> calc plan start and stitch trajectory/10(pre_trajectory_heading)
  [pre_trajectory_x] -> calc plan start and stitch trajectory/8(pre_trajectory_x)
  [host_ay] -> calc plan start and stitch trajectory/7(host_ay)
  [host_ax] -> calc plan start and stitch trajectory/6(host_ax)
  [host_vy] -> calc plan start and stitch trajectory/5(host_vy)
  [host_vx] -> calc plan start and stitch trajectory/4(host_vx)
  [host_heading_xy] -> calc plan start and stitch trajectory/3(host_heading_xy)
  [host_y] -> calc plan start and stitch trajectory/2(host_y)
  [host_x] -> calc plan start and stitch trajectory/1(host_x)
  Bus Selector3/7 -> [pre_trajectory_time]  "<trajectory_time_final[m/s^2]>"
  [trajectory_time_final] -> Bus Creator1/7  "trajectory_time_final[m/s^2]"
  Bus Selector3/5 -> [pre_trajectory_velocity]  "<trajectory_velocity_final[m/s]>"
  Bus Selector3/4 -> [pre_trajectory_kappa]  "<trajectory_kappa_final[1/m]>"
  Bus Selector3/3 -> [pre_trajectory_heading]  "<trajectory_heading_final[rad]>"
  Bus Selector3/2 -> [pre_trajectory_y]  "<trajectory_y_final[m]>"
  Bus Selector3/1 -> [pre_trajectory_x]  "<trajectory_x_final[m]>"
  Bus Selector3/6 -> [pre_trajectory_accelerate]  "<trajectory_accelerate_final[m/s^2]>"
  [planning_info] -> EMplanner_result/1
  Bus Selector/9 -> [host_ay]  "<host_ay>"
  Bus Selector/8 -> [host_ax]  "<host_ax>"
  Selector2/1 -> [origin_y]
  Selector1/1 -> [origin_x]
  Selector/1 -> [origin_match_point_index]
  Bus Selector/7 -> [host_speed]  "<host_speed>"
  Bus Selector/4 -> [host_vx]  "<host_vx>"
  Bus Selector/3 -> [host_heading_xy]  "<host_heading_xy>"
  Bus Selector/6 -> [host_yawrate]  "<host_yawrate>"
  Bus Selector/5 -> [host_vy]  "<host_vy>"
  pre_planning_result/1 -> Bus Selector3/1
  current_time/1 -> [current_time]
  Bus Selector2/4 -> [obs_heading_set_gcs]  "<obs_heading_set_gcs>"
  Bus Selector2/2 -> [obs_y_set_gcs]  "<obs_y_set_gcs>"
  Bus Selector2/3 -> [obs_velocity_set_gcs]  "<obs_velocity_set_gcs>"
  Bus Selector2/1 -> [obs_x_set_gcs]  "<obs_x_set_gcs>"
  perceptiong_result/1 -> Bus Selector2/1
  Bus Selector1/1 -> [referenceline_x]  "<referenceline_x>"
  Bus Selector1/2 -> [referenceline_y]  "<referenceline_y>"
  Bus Selector1/3 -> [referenceline_heading]  "<path_heading>"
  Bus Selector1/4 -> [referenceline_kappa]  "<path_kappa>"
  referenceline_info/1 -> Bus Selector1/1
  Bus Selector/2 -> [host_y]  "<host_y>"
  Location_info/1 -> Bus Selector/1
  Bus Selector/1 -> [host_x]  "<host_x>"
  MATLAB Function1/3(proj_y_set) -> Selector2/1
  [trajectory_kappa_final] -> Bus Creator1/4  "trajectory_kappa_final[1/m]"
  [referenceline_y] -> MATLAB Function1/4(frenet_path_y)
  [trajectory_heading_final] -> Bus Creator1/3  "trajectory_heading_final[rad]"
  [referenceline_heading] -> MATLAB Function1/5(frenet_path_heading)
  MATLAB Function1/5(proj_kappa_set) -> Terminator_2/1
  [referenceline_x] -> MATLAB Function1/3(frenet_path_x)
  [host_y] -> MATLAB Function1/2(y_set)
  MATLAB Function1/1(match_point_index_set) -> Selector/1
  [trajectory_accelerate_final] -> Bus Creator1/6  "trajectory_accelerate_final[m/s^2]"
  Bus Creator1/1 -> [planning_info]
  [host_x] -> MATLAB Function1/1(x_set)
  MATLAB Function1/2(proj_x_set) -> Selector1/1
  [referenceline_kappa] -> MATLAB Function1/6(frenet_path_kappa)
  [trajectory_y_final] -> Bus Creator1/2  "trajectory_y_final[m]"
  [trajectory_x_final] -> Bus Creator1/1  "trajectory_x_final[m]"
  [trajectory_velocity_final] -> Bus Creator1/5  "trajectory_velocity_final[m/s]"
  MATLAB Function1/4(proj_heading_set) -> Terminator_1/1

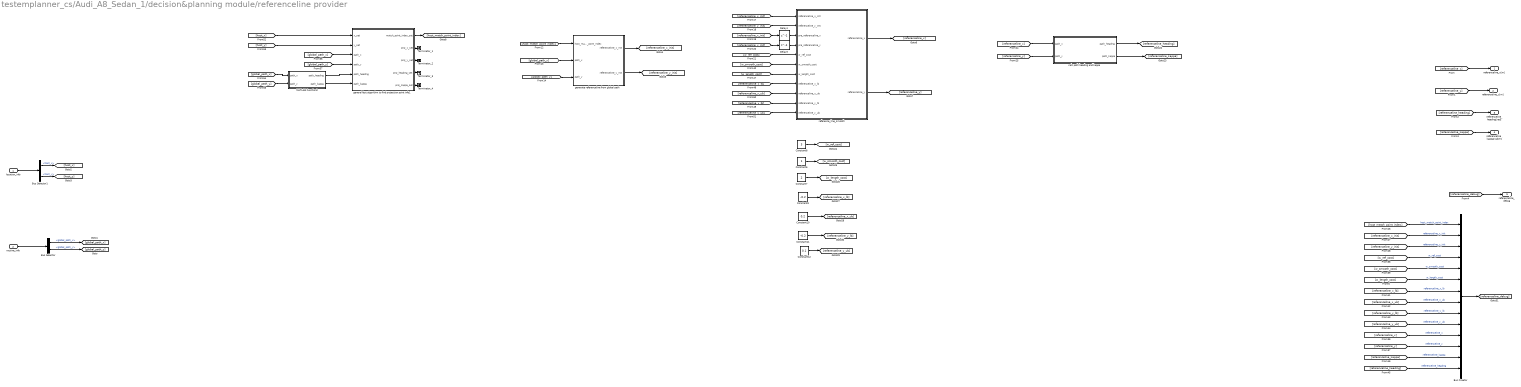
== system testemplanner_cs/Audi_A8_Sedan_1/decision&planning module/referenceline provider ==
  location_info : Inport
  routine_info : Inport  Port=2
  Bus Creator : BusCreator  Inputs=14
  Bus Selector : BusSelector  OutputSignals=global_path_x,global_path_y
  Bus Selector1 : BusSelector  OutputSignals=host_x,host_y
  Constant10 : Constant  Value=0.2
  Constant11 : Constant  Value=-0.2
  Constant12 : Constant  Value=0.1
  Constant6 : Constant
  Constant7 : Constant  Value=2
  Constant8 : Constant  Value=3
  Constant9 : Constant  Value=-0.2
  Delay3 : Delay  DelayLength=1
  Delay4 : Delay  DelayLength=1
  MATLAB Function2 : MATLAB Function  TreatAsAtomicUnit=on
  Terminator_{1..4} (4 alike) : Terminator
  calc path heading and kappa : MATLAB Function  TreatAsAtomicUnit=on
  general fast algorithm to find projection point info1 : MATLAB Function  TreatAsAtomicUnit=on
  generate referenceline from global path : MATLAB Function  TreatAsAtomicUnit=on
  reference_line_smooth : MATLAB Function  TreatAsAtomicUnit=on
  referenceline_x[m] : Outport
  referenceline_y[m] : Outport  Port=2
  referenceline_heading[rad] : Outport  Port=3
  referenceline_kappa[rad/m] : Outport  Port=4
  referenceline_debug : Outport  Port=5
  wires:
  [referenceline_x] -> Bus Creator/11  "referenceline_x"
  [referenceline_heading] -> Bus Creator/14  "referenceline_heading"
  Constant12/1 -> [referenceline_y_ub]
  [referenceline_x_ub] -> Bus Creator/8  "referenceline_x_ub"
  Constant10/1 -> [referenceline_x_ub]
  calc path heading and kappa/1(path_heading) -> [referenceline_heading]
  Constant9/1 -> [referenceline_x_lb]
  [w_ref_cost] -> Bus Creator/4  "w_ref_cost"
  [referenceline_y_lb] -> Bus Creator/9  "referenceline_y_lb"
  Constant6/1 -> [w_smooth_cost]
  calc path heading and kappa/2(path_kappa) -> [referenceline_kappa]
  [referenceline_kappa] -> Bus Creator/13  "referenceline_kappa"
  [referenceline_y_init] -> Bus Creator/3  "referenceline_y_init"
  [referenceline_x_lb] -> Bus Creator/7  "referenceline_x_lb"
  Constant7/1 -> [w_length_cost]
  [w_length_cost] -> Bus Creator/6  "w_length_cost"
  [w_smooth_cost] -> Bus Creator/5  "w_smooth_cost"
  Constant8/1 -> [w_ref_cost]
  Constant11/1 -> [referenceline_y_lb]
  [host_match_point_index] -> Bus Creator/1  "host_match_point_index"
  [referenceline_x_init] -> Bus Creator/2  "referenceline_x_init"
  [referenceline_y] -> Bus Creator/12  "referenceline_y"
  [referenceline_y_ub] -> Bus Creator/10  "referenceline_y_ub"
  Bus Creator/1 -> [referenceline_debug]
  routine_info/1 -> Bus Selector/1
  Bus Selector/2 -> [global_path_y]  "<global_path_y>"
  Bus Selector/1 -> [global_path_x]  "<global_path_x>"
  location_info/1 -> Bus Selector1/1
  Bus Selector1/1 -> [host_x]  "<host_x>"
  Bus Selector1/2 -> [host_y]  "<host_y>"
  [referenceline_kappa] -> referenceline_kappa[rad/m]/1
  [referenceline_heading] -> referenceline_heading[rad]/1
  [referenceline_debug] -> referenceline_debug/1
  [referenceline_x] -> referenceline_x[m]/1
  [referenceline_y] -> referenceline_y[m]/1
  [referenceline_x] -> calc path heading and kappa/1(path_x)
  [referenceline_y] -> calc path heading and kappa/2(path_y)
  [host_match_point_index] -> generate referenceline from global path/1(host_match_point_index)
  [global_path_x] -> generate referenceline from global path/2(path_x)
  [global_path_y] -> generate referenceline from global path/3(path_y)
  generate referenceline from global path/2(referenceline_y_init) -> [referenceline_y_init]
  generate referenceline from global path/1(referenceline_x_init) -> [referenceline_x_init]
  [referenceline_x_init] -> reference_line_smooth/1(referenceline_x_init)
  [referenceline_y_init] -> Delay3/1
  [referenceline_x_init] -> Delay4/1
  [referenceline_y_init] -> reference_line_smooth/2(referenceline_y_init)
  Delay3/1 -> reference_line_smooth/4(pre_referenceline_y)
  Delay4/1 -> reference_line_smooth/3(pre_referenceline_x)
  [w_ref_cost] -> reference_line_smooth/5(w_ref_cost)
  [w_smooth_cost] -> reference_line_smooth/6(w_smooth_cost)
  [w_length_cost] -> reference_line_smooth/7(w_length_cost)
  [referenceline_x_lb] -> reference_line_smooth/8(referenceline_x_lb)
  [referenceline_y_lb] -> reference_line_smooth/10(referenceline_y_lb)
  [referenceline_x_ub] -> reference_line_smooth/9(referenceline_x_ub)
  [referenceline_y_ub] -> reference_line_smooth/11(referenceline_y_ub)
  reference_line_smooth/1(referenceline_x) -> [referenceline_x]
  reference_line_smooth/2(referenceline_y) -> [referenceline_y]
  [global_path_y] -> MATLAB Function2/2(path_y)
  [global_path_x] -> MATLAB Function2/1(path_x)
  general fast algorithm to find projection point info1/4(proj_heading_set) -> Terminator_3/1
  general fast algorithm to find projection point info1/2(proj_x_set) -> Terminator_1/1
  general fast algorithm to find projection point info1/3(proj_y_set) -> Terminator_2/1
  [host_x] -> general fast algorithm to find projection point info1/1(x_set)
  MATLAB Function2/1(path_heading) -> general fast algorithm to find projection point info1/5(path_heading)
  MATLAB Function2/2(path_kappa) -> general fast algorithm to find projection point info1/6(path_kappa)
  [global_path_y] -> general fast algorithm to find projection point info1/4(path_y)
  general fast algorithm to find projection point info1/5(proj_kappa_set) -> Terminator_4/1
  [global_path_x] -> general fast algorithm to find projection point info1/3(path_x)
  general fast algorithm to find projection point info1/1(match_point_index_set) -> [host_match_point_index]
  [host_y] -> general fast algorithm to find projection point info1/2(y_set)

== system testemplanner_cs/Box_1/Dynamics_Empty/MuxState ==
  note: mode: Dynamics
  note: mode: Positioning
  note: mode: Dynamics
      | VelVEHICLE
      | wrt VEH
  note: AnglesVEHICLE
      | wrtGLOB
  note: For state mode 'Dynamic' positions
      | are not taken into account, as they
      | are computed by integrating velocity.
      | Click annotation for Help.
  x [m] : Inport  SampleTime=TimeStep
  y [m] : Inport  Port=2  SampleTime=TimeStep
  z [m] : Inport  Port=3  SampleTime=TimeStep
  dx [m/s] : Inport  Port=4  SampleTime=TimeStep
  dy [m/s] : Inport  Port=5  SampleTime=TimeStep
  dz [m/s] : Inport  Port=6  SampleTime=TimeStep
  R [rad] : Inport  Port=7  SampleTime=TimeStep
  P [rad] : Inport  Port=8  SampleTime=TimeStep
  Y [rad] : Inport  Port=9  SampleTime=TimeStep
  Constant : Constant  DisableCoverage=on  Value=positioningmode
  Discrete-Time Integrator : DiscreteIntegrator  SampleTime=TimeStep  ICPrevOutput=DiscIntNeverNeededParam  ICPrevScaledInput=DiscIntNeverNeededParam
  Ground : Ground
  Ground1 : Ground
  Mux1 : Mux  Inputs=[3 3]
  Mux2 : Mux  Inputs=3
  Mux3 : Mux  Inputs=3
  Mux4 : Mux  Inputs=3
  Mux5 : Mux  Inputs=[3 3]
  Mux6 : Mux  Inputs=[6 3]
  Switch : Switch  Threshold=0.5
  Transformation_BODY2GLOBAL : PreScanSimulinkLibrary/Simple_Vehicle_Dynamics/Chassis/MuxDynState/Transformation_BODY2GLOBAL  SystemSampleTime=-1  Latency=0  AutoFrameSizeCalculation=off
  mux3 : Mux  Inputs=3
  state : Outport
  wires:
  Constant/1 -> Switch/2
  Mux6/1 -> state/1
  Mux4/1 -> Mux1/1
  Mux5/1 -> Switch/3
  Mux1/1 -> Switch/1
  Switch/1 -> Mux6/1  "PosVeh wrt  GLOB"
  P [rad]/1 -> Mux3/2
  R [rad]/1 -> Mux3/1
  dz [m/s]/1 -> Mux2/3
  dy [m/s]/1 -> Mux2/2
  dx [m/s]/1 -> Mux2/1
  z [m]/1 -> Mux4/3
  y [m]/1 -> Mux4/2
  x [m]/1 -> Mux4/1
  Ground1/1 -> mux3/2  "pitch"
  Y [rad]/1 -> mux3/3, Mux3/3  "yaw"
  Mux3/1 -> Mux6/2
  Transformation_BODY2GLOBAL/1 -> Discrete-Time Integrator/1, Mux5/2  "VelVEH wrt  GLOB"
  mux3/1 -> Transformation_BODY2GLOBAL/2
  Ground/1 -> mux3/1  "roll"
  Mux2/1 -> Mux1/2, Transformation_BODY2GLOBAL/1
  Discrete-Time Integrator/1 -> Mux5/1  "PosVEH wrt  GLOB"

== system testemplanner_cs/Box_1/SELF_Demux/compas converter ==
  rotz [rad] : Inport
  cart2compas : Subsystem
  rad2deg : Gain  Gain=180/pi
  heading [deg] : Outport
  wires:
  rad2deg/1 -> cart2compas/1(Angle [deg])
  rotz [rad]/1 -> rad2deg/1
  cart2compas/1(heading [deg]) -> heading [deg]/1

== system testemplanner_cs/Audi_A8_Sedan_1/Dynamics_UserSpecified/CarSim2PreScanSTATE/Transformation_SprungMassCarSim2PreScan ==
  In1 : Inport
  Demux : Demux  Outputs=3
  Ini z-position VEHICLE wrt GLOBAL axis system [m] : Constant  Value=z0
  Mux : Mux  Inputs=3
  Sum1 : Sum  Inputs=+-
  Out1 : Outport
  wires:
  Mux/1 -> Out1/1
  Ini z-position VEHICLE wrt GLOBAL axis system [m]/1 -> Sum1/2
  Demux/1 -> Mux/1
  Sum1/1 -> Mux/3
  Demux/3 -> Sum1/1
  Demux/2 -> Mux/2
  In1/1 -> Demux/1

== system testemplanner_cs/Audi_A8_Sedan_1/SELF_Demux/compas converter/cart2compas ==
  Angle [deg] : Inport
  Constant : Constant  Value=90
  Constant1 : Constant  Value=360
  Gain : Gain  Gain=1/360
  Gain1 : Gain  Gain=360
  Gain2 : Gain  Gain=-1
  Rounding Function : Rounding
  Sum : Sum  Inputs=|-+
  Sum1 : Sum  Inputs=-+|
  Sum2 : Sum  Inputs=++|
  heading [deg] : Outport
  wires:
  Gain/1 -> Rounding Function/1
  Rounding Function/1 -> Gain1/1
  Gain1/1 -> Sum/1
  Angle [deg]/1 -> Sum1/2
  Sum/1 -> Gain2/1
  Sum1/1 -> Gain/1, Sum/2
  Constant/1 -> Sum1/1
  Gain2/1 -> Sum2/2
  Constant1/1 -> Sum2/1
  Sum2/1 -> heading [deg]/1

== system testemplanner_cs/Audi_A8_Sedan_1/Trajectories/Traj2State1/Traj2State2 ==
  traj : Inport
  MuxState : Subsystem
  Traj2MuxState_Ext : Subsystem
  state : Outport
  wires:
  Traj2MuxState_Ext/9(Y [rad]) -> MuxState/9(Y [rad])
  Traj2MuxState_Ext/8(P [rad]) -> MuxState/8(P [rad])
  Traj2MuxState_Ext/7(R [rad]) -> MuxState/7(R [rad])
  Traj2MuxState_Ext/6(dz [m/s]) -> MuxState/6(dz [m/s])
  Traj2MuxState_Ext/5(dy [m/s]) -> MuxState/5(dy [m/s])
  Traj2MuxState_Ext/4(dx [m/s]) -> MuxState/4(dx [m/s])
  Traj2MuxState_Ext/3(z [m]) -> MuxState/3(z [m])
  Traj2MuxState_Ext/2(y [m]) -> MuxState/2(y [m])
  Traj2MuxState_Ext/1(x [m]) -> MuxState/1(x [m])
  MuxState/1(state) -> state/1
  traj/1 -> Traj2MuxState_Ext/1(Traj)

== system testemplanner_cs/Audi_A8_Sedan_1/control module2/control main/chassic steering system ==
  LQR_final_angle : Inport
  Constant : Constant  Value=la
  Constant1 : Constant  Value=lb
  Constant17 : Constant  Value=c_factor
  Divide : Product  Inputs=*/
  Gain3 : Gain  Gain=180/pi
  Gain4 : Gain  Gain=360
  MATLAB Function : MATLAB Function  TreatAsAtomicUnit=on
  Saturation : Saturate  UpperLimit=70  LowerLimit=-70
  Saturation1 : Saturate  UpperLimit=1.2217  LowerLimit=-1.2217
  transfer right wheel angle to rack displancement : Lookup_n-D  NumberOfTableDimensions=1  BreakpointsForDimension1=right_wheel_ground  Table=rack_displacement  InternalRulePriority=Speed  RndMeth=Simplest  InputSameDT=on
  lat_steer_sw[deg] : Outport
  wires:
  MATLAB Function/1(right_steer) -> Gain3/1
  Saturation1/1 -> MATLAB Function/1(u)
  LQR_final_angle/1 -> Saturation1/1
  Constant1/1 -> MATLAB Function/3(lb)
  Gain3/1 -> Saturation/1
  Constant/1 -> MATLAB Function/2(la)
  Saturation/1 -> transfer right wheel angle to rack displancement/1
  Divide/1 -> Gain4/1
  Gain4/1 -> lat_steer_sw[deg]/1
  Constant17/1 -> Divide/2
  transfer right wheel angle to rack displancement/1 -> Divide/1
